simulink subsystem "Studio3_Actuator_Subsystem"  (R2020a)
settings: Solver=VariableStepAuto  StartTime=0.0  StopTime=10.0  RelTol=1e-3
libraries: Studio3_Actuator_library x1
settings Model: Creator=ethoma  LastModifiedBy=Emily

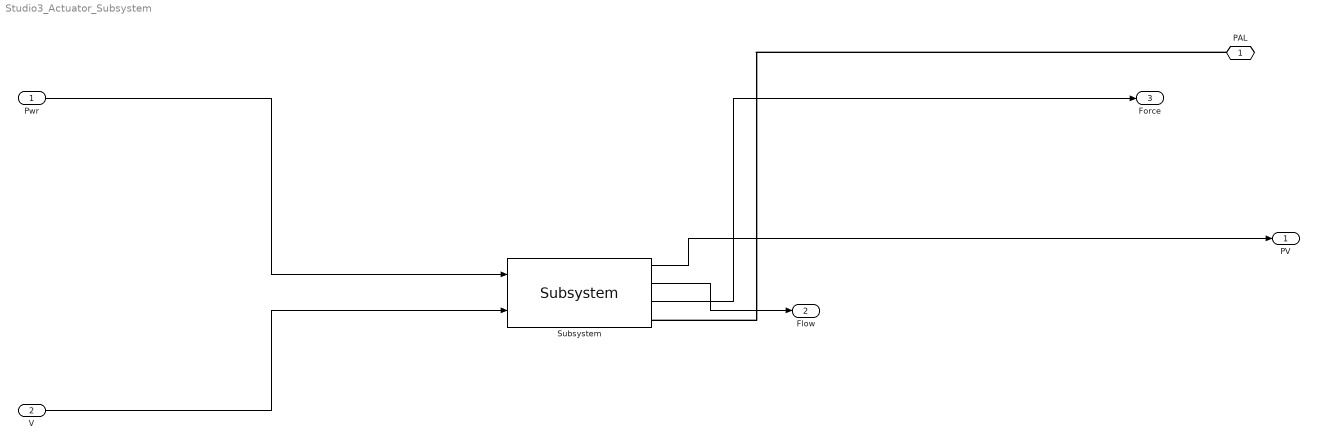
== system Studio3_Actuator_Subsystem ==
  Pwr : Inport
  V : Inport  Port=2
  Subsystem : Studio3_Actuator_library/Subsystem  SystemSampleTime=-1  Latency=0  AutoFrameSizeCalculation=off
  PAL : PMIOPort  Side=Left
  PV : Outport
  Flow : Outport  Port=2
  Force : Outport  Port=3
  wires:
  Pwr/1 -> Subsystem/1
  V/1 -> Subsystem/2
  Subsystem/1 -> PV/1
  Subsystem/2 -> Flow/1
  Subsystem/3 -> Force/1
  connections:
  PAL/RConn1 -- Subsystem/RConn1
